simulink model "AmplitudeModulation"  (R2018a)
settings: Solver=VariableStepAuto  StartTime=0.0  StopTime=0.005  RelTol=1e-3
settings Model: Creator=Neo  LastModifiedBy=Neo

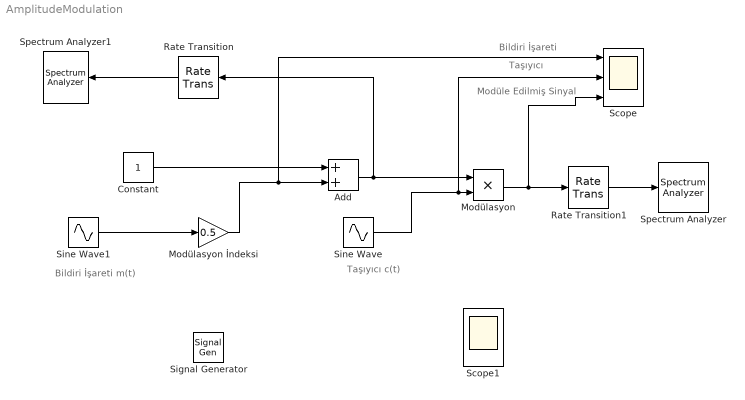
== system AmplitudeModulation ==
  note: Taşıyıcı
      | c(t)
  note: Bildiri İşareti
      | 	m(t)
  note: Modüle Edilmiş Sinyal
  note: Taşıyıcı
  note: Bildiri İşareti
  Add : Sum
  Constant : Constant
  Modülasyon : Product
  Modülasyon İndeksi : Gain  Gain=0.5
  Rate Transition : RateTransition  OutPortSampleTime=1/8e4
  Rate Transition1 : RateTransition  OutPortSampleTime=1/8e4
  Scope : Scope  NumInputPorts=3
  Scope1 : Scope  NumInputPorts=2
  Signal Generator : SignalGenerator  WaveForm=square  Frequency=1000
  Sine Wave : Sin  Frequency=2*pi*10000  Phase=pi/2  SampleTime=0
  Sine Wave1 : Sin  Frequency=2*pi*1000  SampleTime=0
  Spectrum Analyzer : SpectrumAnalyzer
  Spectrum Analyzer1 : SpectrumAnalyzer
  wires:
  Rate Transition/1 -> Spectrum Analyzer1/1
  Add/1 -> Rate Transition/1, Modülasyon/1
  Modülasyon İndeksi/1 -> Scope/1, Add/2
  Rate Transition1/1 -> Spectrum Analyzer/1
  Modülasyon/1 -> Rate Transition1/1, Scope/3
  Constant/1 -> Add/1
  Sine Wave/1 -> Scope/2, Modülasyon/2
  Sine Wave1/1 -> Modülasyon İndeksi/1
